simulink model "motor_1_2_3"  (R2023a)
settings: Solver=ode15s  StartTime=0.0  StopTime=sim_end_time  MaxStep=sim_max_step  RelTol=1e-3
values from neighbouring files (symbols this model uses):
  alpha_cu = 3.9 *10^-3    (= 0.0039)    [BLDC_Motor_params_03.m]    (also in DC_Motor_params_01.m; DC_Motor_params_02.m; DC_Motor_params_04.m; DC_Motor_params_05.m)
  b_m1 = .01    (= 0.01)    [DC_Motor_params_01.m]
  b_m2 = .01    (= 0.01)    [DC_Motor_params_02.m]
  b_m3 = .001    (= 0.001)    [BLDC_Motor_params_03.m]
  C_t1 = 19.57    [DC_Motor_params_01.m]
  C_t2 = 66.49    [DC_Motor_params_02.m]
  C_t3 = 50    [BLDC_Motor_params_03.m]
  ENABLE_SATURATIONS = 1    [run_flags.m]
  ENABLE_SENSORS = 1    [run_flags.m]
  enc_ppr_1 = 1024    [DC_Motor_params_01.m]
  enc_ppr_2 = 1024    [DC_Motor_params_02.m]
  filter_RC = 1/(max_freq*2*pi)    (= 0.00795774715459)    [filter_params.m]
  J_eq1 = J_1 + 1/8 * m_1 * d_1^2 / r_1^2    [DC_Motor_params_01.m]
  J_eq2 = J_2 + 1/8 * m_2 * d_2^2 / r_2^2    [DC_Motor_params_02.m]
  J_eq3 = J_3 + 1/8 * m_3 * d_3^2 / r_3^2    [BLDC_Motor_params_03.m]
  K_d1 = 0.022261    [PID_tuning.m]
  K_d2 = 0.07064    [PID_tuning.m]
  K_d3 = 0    [PID_tuning.m]
  k_e1 = 0.25    [DC_Motor_params_01.m]
  k_e2 = 0.56    [DC_Motor_params_02.m]
  k_e3 = 0.3    [BLDC_Motor_params_03.m]
  K_i1 = 0    [PID_tuning.m]
  K_i2 = 0    [PID_tuning.m]
  K_i3 = 0.4131    [PID_tuning.m]
  K_p1 = 6.6674    [PID_tuning.m]
  K_p2 = 15.5368    [PID_tuning.m]
  K_p3 = 0    [PID_tuning.m]
  k_t1 = 0.25    [DC_Motor_params_01.m]
  k_t2 = 0.56    [DC_Motor_params_02.m]
  k_t3 = 0.3    [BLDC_Motor_params_03.m]
  L_a1 = 7.5*10^-3    (= 0.0075)    [DC_Motor_params_01.m]
  L_a2 = 3*10^-3    (= 0.003)    [DC_Motor_params_02.m]
  L_a3 = 5*10^-3    (= 0.005)    [BLDC_Motor_params_03.m]
  r_1 = 25    [DC_Motor_params_01.m]
  r_2 = 5    [DC_Motor_params_02.m]
  r_3 = 2    [BLDC_Motor_params_03.m]
  r_a1_20 = 0.5    [DC_Motor_params_01.m]
  r_a2_20 = 0.25    [DC_Motor_params_02.m]
  r_a3_20 = 0.35    [BLDC_Motor_params_03.m]
  res_term_1 = 9.58    [DC_Motor_params_01.m]
  res_term_2 = 3.15    [DC_Motor_params_02.m]
  res_term_3 = 0.1    [BLDC_Motor_params_03.m]
  sampling_frequency = 40    [filter_params.m]
  T_s0_1 = 20    [use_machine_1.m]    (also in use_solo_motor_1.m)
  T_s0_2 = 20    [use_machine_1.m]    (also in use_solo_motor_2.m)
  T_s0_3 = 20    [use_machine_1.m]    (also in use_solo_motor_3.m)
  theta_m0_1 = 0    [use_machine_1.m]    (also in use_solo_motor_1.m)
  theta_m0_2 = 0    [use_machine_1.m]    (also in use_solo_motor_2.m = 3.14159265359)
  voltage_1 = 12    [DC_Motor_params_01.m]
  voltage_2 = 110    [DC_Motor_params_02.m]
  voltage_3 = 220    [BLDC_Motor_params_03.m]
libraries: slpidlib x1
settings Model: Creator=Usuario  LastModifiedBy=Usuario
settings DataIOCC: ExternalInput=[sim_t, sim_data_in]  LoadExternalInput=on

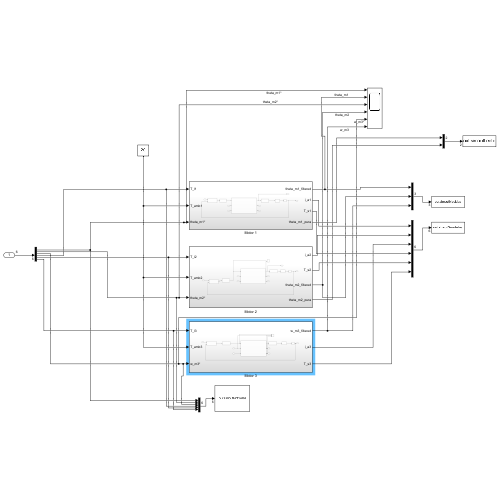
[thumbnail: Simulink's stored preview of the top-level diagram]
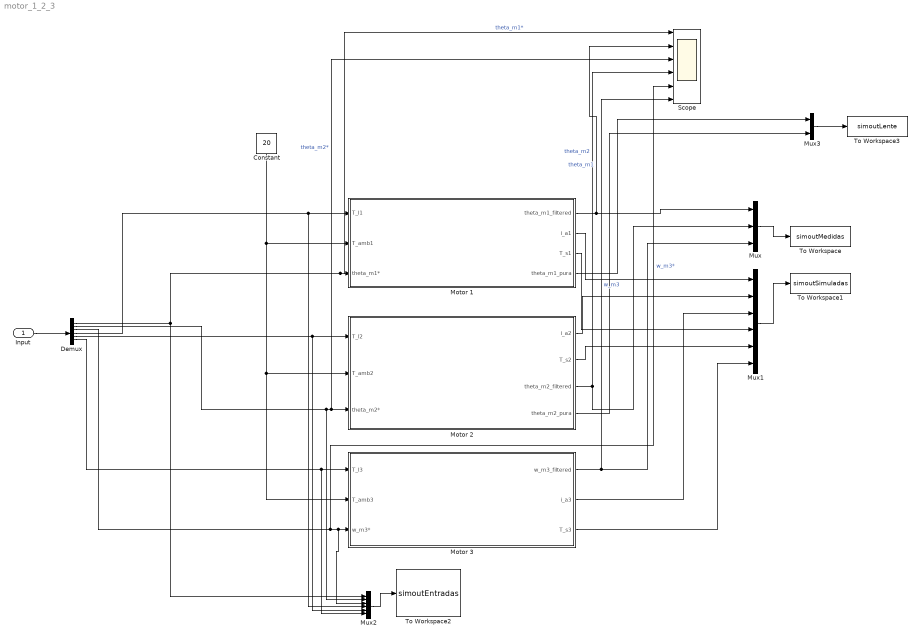
== system motor_1_2_3 ==
  Input : Inport
  Constant : Constant  Value=20
  Demux : Demux  Outputs=6
  Motor 1 : Subsystem
  Motor 2 : Subsystem
  Motor 3 : Subsystem
  Mux : Mux  Inputs=3
  Mux1 : Mux  Inputs=6
  Mux2 : Mux  Inputs=6
  Mux3 : Mux  Inputs=2
  Scope : Scope  NumInputPorts=6
  To Workspace : ToWorkspace  VariableName=simoutMedidas  SaveFormat=Timeseries  SampleTime=-1
  To Workspace1 : ToWorkspace  VariableName=simoutSimuladas  SaveFormat=Timeseries  SampleTime=-1
  To Workspace2 : ToWorkspace  VariableName=simoutEntradas  SaveFormat=Timeseries  SampleTime=-1
  To Workspace3 : ToWorkspace  VariableName=simoutLente  SaveFormat=Timeseries  SampleTime=-1
  wires:
  Constant/1 -> Motor 3/2(T_amb3), Motor 2/2(T_amb2), Motor 1/2(T_amb1)
  Input/1 -> Demux/1
  Demux/2 -> Mux2/2, Scope/3, Motor 2/3(theta_m2*)  "theta_m2*"
  Demux/3 -> Scope/5, Mux2/3, Motor 3/3(w_m3*)  "w_m3*"
  Demux/4 -> Mux2/4, Motor 1/1(T_l1)
  Demux/5 -> Mux2/5, Motor 2/1(T_l2)
  Demux/6 -> Mux2/6, Motor 3/1(T_l3)
  Demux/1 -> Scope/1, Motor 1/3(theta_m1*), Mux2/1  "theta_m1*"
  Motor 2/3(theta_m2_filtered) -> Mux/2, Scope/4  "theta_m2"
  Motor 3/1(w_m3_filtered) -> Scope/6, Mux/3  "w_m3"
  Motor 1/2(i_a1) -> Mux1/1
  Motor 2/1(i_a2) -> Mux1/2
  Motor 3/2(i_a3) -> Mux1/3
  Motor 1/3(T_s1) -> Mux1/4
  Motor 2/2(T_s2) -> Mux1/5
  Motor 3/3(T_s3) -> Mux1/6
  Mux/1 -> To Workspace/1
  Mux1/1 -> To Workspace1/1
  Motor 1/1(theta_m1_filtered) -> Scope/2, Mux/1  "theta_m1"
  Mux2/1 -> To Workspace2/1
  Mux3/1 -> To Workspace3/1
  Motor 1/4(theta_m1_pura) -> Mux3/1
  Motor 2/4(theta_m2_pura) -> Mux3/2

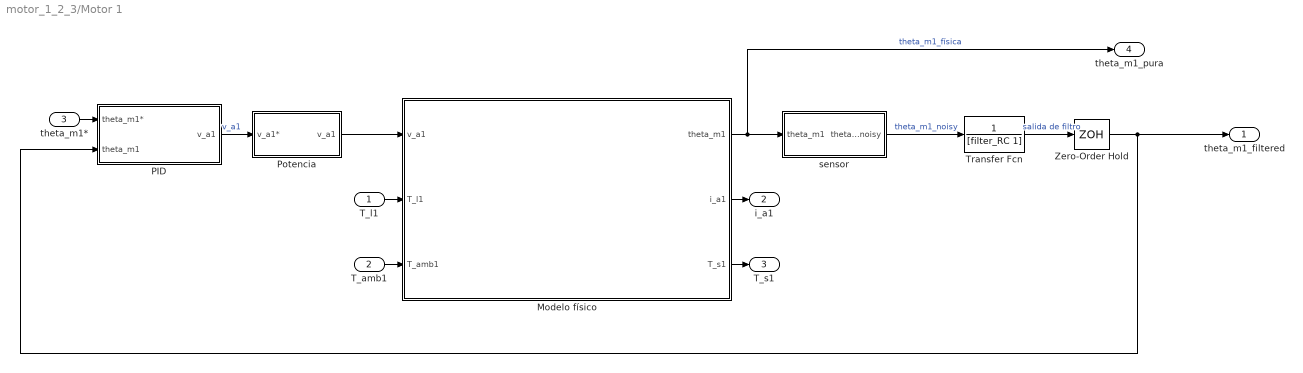
== system motor_1_2_3/Motor 1 ==
  T_l1 : Inport
  T_amb1 : Inport  Port=2
  theta_m1* : Inport  Port=3
  Modelo físico : Subsystem
  PID : Subsystem
  Potencia : Subsystem
  Transfer Fcn : TransferFcn  Denominator=[filter_RC 1]
  Zero-Order Hold : ZeroOrderHold  SampleTime=1/sampling_frequency
  sensor : Subsystem
  theta_m1_filtered : Outport  PortDimensions=1
  i_a1 : Outport  Port=2  PortDimensions=1
  T_s1 : Outport  Port=3  PortDimensions=1
  theta_m1_pura : Outport  Port=4
  wires:
  Modelo físico/1(theta_m1) -> theta_m1_pura/1, sensor/1(theta_m1)  "theta_m1_física"
  theta_m1*/1 -> PID/1(theta_m1*)
  Zero-Order Hold/1 -> PID/2(theta_m1), theta_m1_filtered/1
  sensor/1(theta_m1_noisy) -> Transfer Fcn/1  "theta_m1_noisy"
  Potencia/1(v_a1) -> Modelo físico/1(v_a1)
  Modelo físico/2(i_a1) -> i_a1/1
  Modelo físico/3(T_s1) -> T_s1/1
  T_amb1/1 -> Modelo físico/3(T_amb1)
  T_l1/1 -> Modelo físico/2(T_l1)
  PID/1(v_a1) -> Potencia/1(v_a1*)  "v_a1"
  Transfer Fcn/1 -> Zero-Order Hold/1  "salida de filtro"

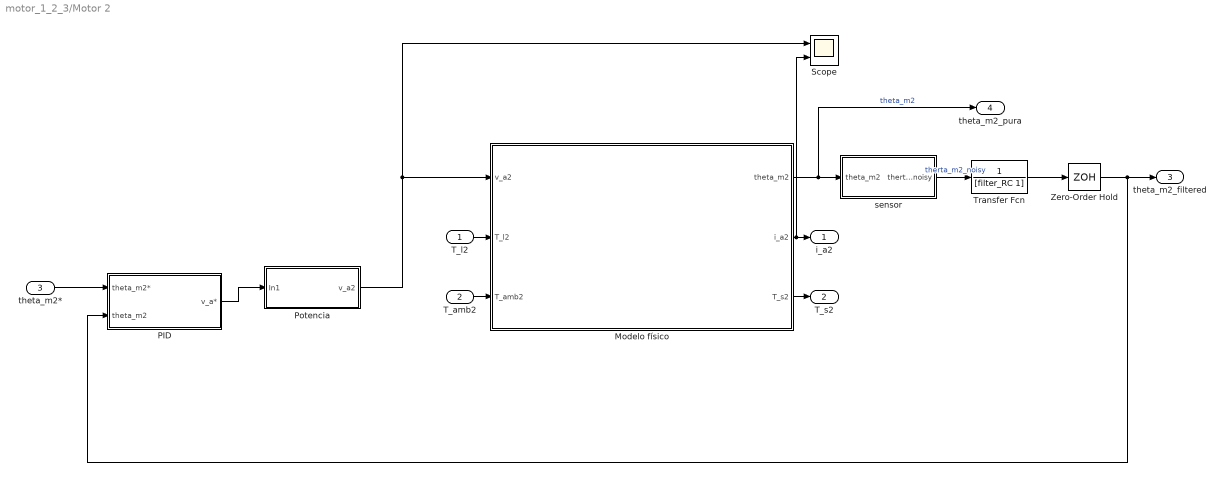
== system motor_1_2_3/Motor 2 ==
  T_l2 : Inport
  T_amb2 : Inport  Port=2
  theta_m2* : Inport  Port=3
  Modelo físico : Subsystem
  PID : Subsystem
  Potencia : Subsystem
  Scope : Scope  NumInputPorts=2
  Transfer Fcn : TransferFcn  Denominator=[filter_RC 1]
  Zero-Order Hold : ZeroOrderHold  SampleTime=1/sampling_frequency
  sensor : Subsystem
  i_a2 : Outport  PortDimensions=1
  T_s2 : Outport  Port=2  PortDimensions=1
  theta_m2_filtered : Outport  Port=3  PortDimensions=1
  theta_m2_pura : Outport  Port=4
  wires:
  sensor/1(therta_m2_noisy) -> Transfer Fcn/1  "therta_m2_noisy"
  Modelo físico/2(i_a2) -> Scope/2, i_a2/1
  Zero-Order Hold/1 -> theta_m2_filtered/1, PID/2(theta_m2)
  T_amb2/1 -> Modelo físico/3(T_amb2)
  T_l2/1 -> Modelo físico/2(T_l2)
  Potencia/1(v_a2) -> Scope/1, Modelo físico/1(v_a2)
  theta_m2*/1 -> PID/1(theta_m2*)
  Modelo físico/3(T_s2) -> T_s2/1
  PID/1(v_a*) -> Potencia/1(In1)
  Modelo físico/1(theta_m2) -> theta_m2_pura/1, sensor/1(theta_m2)  "theta_m2"
  Transfer Fcn/1 -> Zero-Order Hold/1

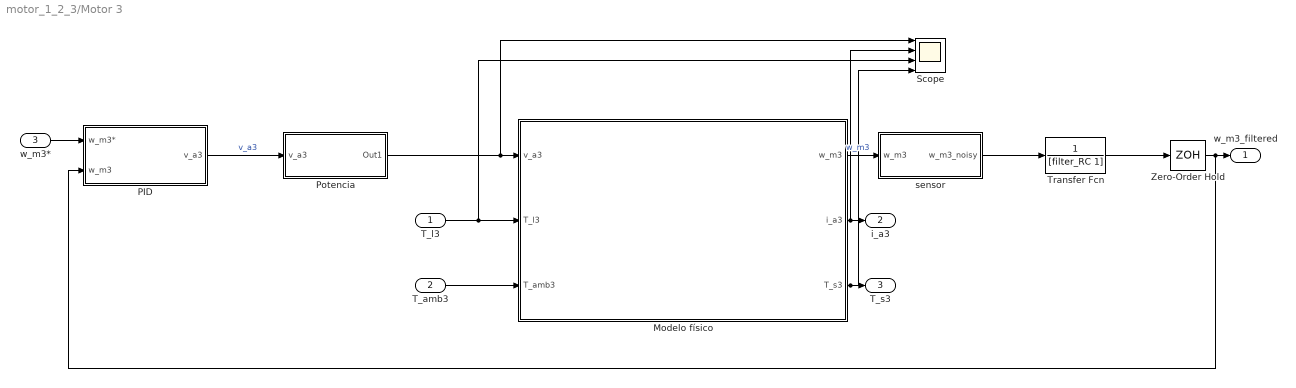
== system motor_1_2_3/Motor 3 ==
  T_l3 : Inport
  T_amb3 : Inport  Port=2
  w_m3* : Inport  Port=3
  Modelo físico : Subsystem
  PID : Subsystem
  Potencia : Subsystem
  Scope : Scope  NumInputPorts=4
  Transfer Fcn : TransferFcn  Denominator=[filter_RC 1]
  Zero-Order Hold : ZeroOrderHold  SampleTime=1/sampling_frequency
  sensor : Subsystem
  w_m3_filtered : Outport
  i_a3 : Outport  Port=2
  T_s3 : Outport  Port=3
  wires:
  PID/1(v_a3) -> Potencia/1(v_a3)  "v_a3"
  T_amb3/1 -> Modelo físico/3(T_amb3)
  sensor/1(w_m3_noisy) -> Transfer Fcn/1
  Potencia/1(Out1) -> Scope/1, Modelo físico/1(v_a3)
  T_l3/1 -> Scope/3, Modelo físico/2(T_l3)
  Modelo físico/1(w_m3) -> sensor/1(w_m3)  "w_m3"
  Modelo físico/3(T_s3) -> Scope/4, T_s3/1
  Zero-Order Hold/1 -> PID/2(w_m3), w_m3_filtered/1
  Modelo físico/2(i_a3) -> Scope/2, i_a3/1
  w_m3*/1 -> PID/1(w_m3*)
  Transfer Fcn/1 -> Zero-Order Hold/1

== system motor_1_2_3/Motor 1/Modelo físico ==
  v_a1 : Inport
  T_l1 : Inport  Port=2
  T_amb1 : Inport  Port=3
  Subsistema electromagnético : Subsystem
  Subsistema mecánico : Subsystem
  Subsistema térmico : Subsystem
  theta_m1 : Outport
  i_a1 : Outport  Port=2  PortDimensions=1
  T_s1 : Outport  Port=3  PortDimensions=1
  wires:
  Subsistema electromagnético/1(i_a1) -> Subsistema térmico/1(i_a1), Subsistema mecánico/1(i_a1), i_a1/1
  v_a1/1 -> Subsistema electromagnético/1(v_a1)
  T_l1/1 -> Subsistema mecánico/2(T_l1)
  T_amb1/1 -> Subsistema térmico/2(T_amb1)
  Subsistema térmico/1(T_s1) -> T_s1/1
  Subsistema térmico/2(r_a1) -> Subsistema electromagnético/2(r_a1)
  Subsistema mecánico/1(w_m1) -> Subsistema electromagnético/3(w_m1)
  Subsistema mecánico/2(theta_m1) -> theta_m1/1

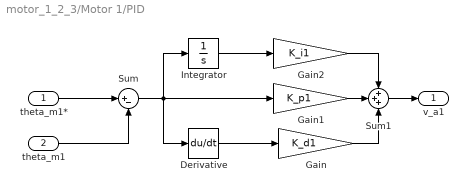
== system motor_1_2_3/Motor 1/PID ==
  theta_m1* : Inport
  theta_m1 : Inport  Port=2
  Derivative : Derivative
  Gain : Gain  Gain=K_d1
  Gain1 : Gain  Gain=K_p1
  Gain2 : Gain  Gain=K_i1
  Integrator : Integrator
  Sum : Sum  Inputs=|+-
  Sum1 : Sum  Inputs=+++
  v_a1 : Outport
  wires:
  theta_m1*/1 -> Sum/1
  theta_m1/1 -> Sum/2
  Sum/1 -> Integrator/1, Gain1/1, Derivative/1
  Integrator/1 -> Gain2/1
  Derivative/1 -> Gain/1
  Gain1/1 -> Sum1/2
  Gain2/1 -> Sum1/1
  Sum1/1 -> v_a1/1
  Gain/1 -> Sum1/3

== system motor_1_2_3/Motor 1/Potencia ==
  v_a1* : Inport
  Gain : Gain  Gain=ENABLE_SATURATIONS
  Gain1 : Gain  Gain=1-ENABLE_SATURATIONS
  Saturation : Saturate  UpperLimit=+voltage_1  LowerLimit=-voltage_1
  Sum : Sum  Inputs=|++
  v_a1 : Outport
  wires:
  v_a1*/1 -> Gain1/1, Saturation/1
  Saturation/1 -> Gain/1
  Gain/1 -> Sum/1
  Sum/1 -> v_a1/1
  Gain1/1 -> Sum/2

== system motor_1_2_3/Motor 1/sensor ==
  theta_m1 : Inport
  Gain : Gain  Gain=ENABLE_SENSORS
  Gain1 : Gain  Gain=1-ENABLE_SENSORS
  Scope : Scope  NumInputPorts=2
  Sum : Sum  Inputs=++|
  ruido de cuantización : Quantizer  QuantizationInterval=360/enc_ppr_1*(pi/180)
  theta_m1_noisy : Outport
  wires:
  Gain/1 -> Sum/2
  Gain1/1 -> Sum/1
  ruido de cuantización/1 -> Gain/1, Scope/1
  theta_m1/1 -> Gain1/1, ruido de cuantización/1, Scope/2
  Sum/1 -> theta_m1_noisy/1

== system motor_1_2_3/Motor 2/Modelo físico ==
  v_a2 : Inport
  T_l2 : Inport  Port=2
  T_amb2 : Inport  Port=3
  Subsistema electromagnético : Subsystem
  Subsistema mecánico : Subsystem
  Subsistema térmico : Subsystem
  theta_m2 : Outport
  i_a2 : Outport  Port=2  PortDimensions=1
  T_s2 : Outport  Port=3  PortDimensions=1
  wires:
  Subsistema electromagnético/1(i_a2) -> Subsistema térmico/1(i_a2), Subsistema mecánico/1(i_a2), i_a2/1
  v_a2/1 -> Subsistema electromagnético/1(v_a2)
  T_l2/1 -> Subsistema mecánico/2(T_l2)
  T_amb2/1 -> Subsistema térmico/2(T_amb2)
  Subsistema térmico/1(T_s2) -> T_s2/1
  Subsistema térmico/2(r_a2) -> Subsistema electromagnético/2(r_a2)
  Subsistema mecánico/1(w_m2) -> Subsistema electromagnético/3(w_m2)
  Subsistema mecánico/2(theta_m2) -> theta_m2/1

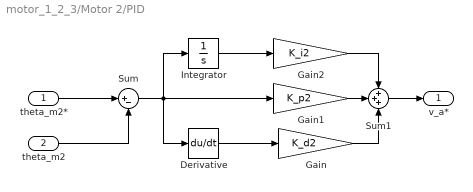
== system motor_1_2_3/Motor 2/PID ==
  theta_m2* : Inport
  theta_m2 : Inport  Port=2
  Derivative : Derivative
  Gain : Gain  Gain=K_d2
  Gain1 : Gain  Gain=K_p2
  Gain2 : Gain  Gain=K_i2
  Integrator : Integrator
  Sum : Sum  Inputs=|+-
  Sum1 : Sum  Inputs=+++
  v_a* : Outport
  wires:
  theta_m2*/1 -> Sum/1
  theta_m2/1 -> Sum/2
  Sum/1 -> Integrator/1, Gain1/1, Derivative/1
  Integrator/1 -> Gain2/1
  Derivative/1 -> Gain/1
  Gain1/1 -> Sum1/2
  Gain2/1 -> Sum1/1
  Sum1/1 -> v_a*/1
  Gain/1 -> Sum1/3

== system motor_1_2_3/Motor 2/Potencia ==
  In1 : Inport
  Gain : Gain  Gain=ENABLE_SATURATIONS
  Gain1 : Gain  Gain=1-ENABLE_SATURATIONS
  Saturation : Saturate  UpperLimit=+voltage_2  LowerLimit=-voltage_2
  Sum : Sum  Inputs=++|
  v_a2 : Outport
  wires:
  Saturation/1 -> Sum/2
  Gain/1 -> Saturation/1
  In1/1 -> Gain1/1, Gain/1
  Sum/1 -> v_a2/1
  Gain1/1 -> Sum/1

== system motor_1_2_3/Motor 2/sensor ==
  theta_m2 : Inport
  Gain : Gain  Gain=ENABLE_SENSORS
  Gain1 : Gain  Gain=1-ENABLE_SENSORS
  Scope : Scope  NumInputPorts=2
  Sum : Sum  Inputs=++|
  ruido de cuantización : Quantizer  QuantizationInterval=360/enc_ppr_2*(pi/180)
  therta_m2_noisy : Outport
  wires:
  Gain/1 -> Sum/2
  Gain1/1 -> Sum/1
  ruido de cuantización/1 -> Gain/1, Scope/1
  theta_m2/1 -> Gain1/1, ruido de cuantización/1, Scope/2
  Sum/1 -> therta_m2_noisy/1

== system motor_1_2_3/Motor 3/Modelo físico ==
  v_a3 : Inport
  T_l3 : Inport  Port=2
  T_amb3 : Inport  Port=3
  Subsistema electromagnético : Subsystem
  Subsistema mecánico : Subsystem
  Subsistema térmico : Subsystem
  w_m3 : Outport  PortDimensions=1
  i_a3 : Outport  Port=2  PortDimensions=1
  T_s3 : Outport  Port=3  PortDimensions=1
  wires:
  Subsistema electromagnético/1(i_a3) -> Subsistema térmico/1(i_a3), Subsistema mecánico/1(i_a3), i_a3/1
  v_a3/1 -> Subsistema electromagnético/1(v_a3)
  T_l3/1 -> Subsistema mecánico/2(T_l3)
  Subsistema mecánico/1(w_m3) -> w_m3/1, Subsistema electromagnético/3(w_m3)
  T_amb3/1 -> Subsistema térmico/2(T_amb3)
  Subsistema térmico/1(T_s3) -> T_s3/1
  Subsistema térmico/2(r_a3) -> Subsistema electromagnético/2(r_a3)

== system motor_1_2_3/Motor 3/PID ==
  w_m3* : Inport
  w_m3 : Inport  Port=2
  PID Controller : slpidlib/PID Controller  Controller=PID  Form=Parallel  TimeDomain=Continuous-time  UseExternalTs=off  SampleTime=-1  IntegratorMethod=Forward Euler  FilterMethod=Forward Euler  ControllerParametersSource=internal  P=K_p3  I=K_i3  UseKiTs=off  D=K_d3  N=100  UseFilter=on  TunerSelectOption=Transfer Function Based (PID Tuner App)  InitialConditionSource=internal  InitialConditionForIntegrator=0  InitialConditionForFilter=0  DifferentiatorICPrevScaledInput=0  ExternalReset=none  TrackingMode=off  Kt=1  LimitOutput=on  SatLimitsSource=internal  UpperSaturationLimit=voltage_3  LowerSaturationLimit=-voltage_3  LinearizeAsGain=on  AntiWindupMode=back-calculation  Kb=K_i3  LimitIntegrator=off  UpperIntegratorSaturationLimit=inf  LowerIntegratorSaturationLimit=-inf  POutMin=[]  POutMax=[]  IOutMin=[]  IOutMax=[]  DOutMin=[]  DOutMax=[]  NOutMin=[]  NOutMax=[]  SumOutMin=[]  SumOutMax=[]  SaturationOutMin=[]  SaturationOutMax=[]  PParamMin=[]  PParamMax=[]  IParamMin=[]  IParamMax=[]  DParamMin=[]  DParamMax=[]  NParamMin=[]  NParamMax=[]  KbParamMin=[]  KbParamMax=[]  KtParamMin=[]  KtParamMax=[]  KbOutMin=[]  KbOutMax=[]  KtOutMin=[]  KtOutMax=[]  IntegratorOutMin=[]  IntegratorOutMax=[]  FilterOutMin=[]  FilterOutMax=[]  SumI1OutMin=[]  SumI1OutMax=[]  SumI2OutMin=[]  SumI2OutMax=[]  SumI3OutMin=[]  SumI3OutMax=[]  SumI4OutMin=[]  SumI4OutMax=[]  SumDOutMin=[]  SumDOutMax=[]  DifferentiatorOutMin=[]  DifferentiatorOutMax=[]  FilterDiffOutCoefMin=[]  FilterDiffOutCoefMax=[]  ReciprocalOutMin=[]  ReciprocalOutMax=[]  SumDenOutMin=[]  SumDenOutMax=[]  SumNumOutMin=[]  SumNumOutMax=[]  DivideOutMin=[]  DivideOutMax=[]  UdiffTsProdOutMin=[]  UdiffTsProdOutMax=[]  NTsProdOutMin=[]  NTsProdOutMax=[]  UintegralTsProdOutMin=[]  UintegralTsProdOutMax=[]  UngainTsProdOutMin=[]  UngainTsProdOutMax=[]  ClampingZeroOutDataTypeStr=Inherit: Inherit via back propagation  ClampingZeroOutMin=[]  ClampingZeroOutMax=[]  FilterDenConstantOutDataTypeStr=Inherit: Inherit via back propagation  FilterDenConstantOutMin=[]  FilterDenConstantOutMax=[]  PCopyOutDataTypeStr=Inherit: Inherit via back propagation  PCopyOutMin=[]  PCopyOutMax=[]  NCopyOutDataTypeStr=Inherit: Inherit via back propagation  NCopyOutMin=[]  NCopyOutMax=[]  IntegratorContinuousStateAttributes=''  IntegratorStateMustResolveToSignalObject=off  IntegratorRTWStateStorageClass=Auto  FilterContinuousStateAttributes=''  FilterStateMustResolveToSignalObject=off  FilterRTWStateStorageClass=Auto  ParallelPVariant=InternalParameters  IdealPVariant=Disabled  IVariant=InternalParameters  DVariant=InternalParameters  IntegratorVariant=Continuous  SatVariant=Enabled  AWVariant=BackCalculation  PCopyVariant=Disabled  TRVariant=Disabled  FdbkBlocksVariant=Forward  IdealPFdbkVariant=Disabled  SatFdbkVariant=Disabled  DerivativeFilterVariant=ContFilter  NVariant=InternalParameters  NCopyVariant=Disabled  FilterICVariant=InternalICsFilter  IntegratorICVariant=InternalICs  ExternalResetVariant=Disabled  TRSumVariant=Passthrough  SumFdbkVariant=Disabled  SumVariant=Sum_PID  TsampFilterVariant=InternalTs  TsampNgainVariant=Passthrough  TsampIntegralVariant=Disabled_SignalSpec  ExternalSaturationOutDataTypeStr=Inherit: Same as second input
  Sum : Sum  Inputs=|+-
  v_a3 : Outport
  wires:
  w_m3*/1 -> Sum/1
  w_m3/1 -> Sum/2
  Sum/1 -> PID Controller/1
  PID Controller/1 -> v_a3/1

== system motor_1_2_3/Motor 3/Potencia ==
  v_a3 : Inport
  Gain : Gain  Gain=ENABLE_SATURATIONS
  Gain1 : Gain  Gain=1-ENABLE_SATURATIONS
  Saturation : Saturate  UpperLimit=+voltage_3  LowerLimit=-voltage_3
  Sum : Sum  Inputs=++|
  Out1 : Outport
  wires:
  v_a3/1 -> Gain1/1, Gain/1
  Saturation/1 -> Sum/2
  Gain/1 -> Saturation/1
  Sum/1 -> Out1/1
  Gain1/1 -> Sum/1

== system motor_1_2_3/Motor 3/sensor ==
  w_m3 : Inport
  Gain : Gain  Gain=1/(2*pi)
  Gain1 : Gain  Gain=(2*pi)
  Gain2 : Gain  Gain=ENABLE_SENSORS
  Gain3 : Gain  Gain=1-ENABLE_SENSORS
  Quantizer : Quantizer  QuantizationInterval=sensibilidad_sensor_3
  Scope : Scope  NumInputPorts=2
  Sum : Sum  Inputs=++|
  w_m3_noisy : Outport
  wires:
  w_m3/1 -> Gain3/1, Gain2/1
  Quantizer/1 -> Gain1/1, Scope/1
  Gain/1 -> Quantizer/1
  Gain1/1 -> Sum/2
  Gain2/1 -> Scope/2, Gain/1
  Gain3/1 -> Sum/1
  Sum/1 -> w_m3_noisy/1

== system motor_1_2_3/Motor 1/Modelo físico/Subsistema electromagnético ==
  v_a1 : Inport
  r_a1 : Inport  Port=2
  w_m1 : Inport  Port=3
  Gain1 : Gain  Gain=k_e1
  Gain2 : Gain  Gain=1/L_a1
  Integrator : Integrator
  Product : Product
  Sum : Sum  Inputs=-+-  OutMin=[1]  OutMax=[1]
  i_a1 : Outport
  wires:
  v_a1/1 -> Sum/2
  Integrator/1 -> Product/2, i_a1/1
  Product/1 -> Sum/1
  w_m1/1 -> Gain1/1
  Gain1/1 -> Sum/3
  Sum/1 -> Gain2/1
  Gain2/1 -> Integrator/1
  r_a1/1 -> Product/1

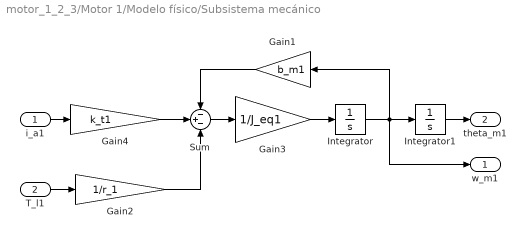
== system motor_1_2_3/Motor 1/Modelo físico/Subsistema mecánico ==
  i_a1 : Inport
  T_l1 : Inport  Port=2
  Gain1 : Gain  Gain=b_m1
  Gain2 : Gain  Gain=1/r_1
  Gain3 : Gain  Gain=1/J_eq1
  Gain4 : Gain  Gain=k_t1
  Integrator : Integrator
  Integrator1 : Integrator  InitialCondition=theta_m0_1
  Sum : Sum  Inputs=-+-
  w_m1 : Outport
  theta_m1 : Outport  Port=2
  wires:
  i_a1/1 -> Gain4/1
  Integrator/1 -> w_m1/1, Gain1/1, Integrator1/1
  Gain1/1 -> Sum/1
  T_l1/1 -> Gain2/1
  Gain3/1 -> Integrator/1
  Sum/1 -> Gain3/1
  Integrator1/1 -> theta_m1/1
  Gain2/1 -> Sum/3
  Gain4/1 -> Sum/2

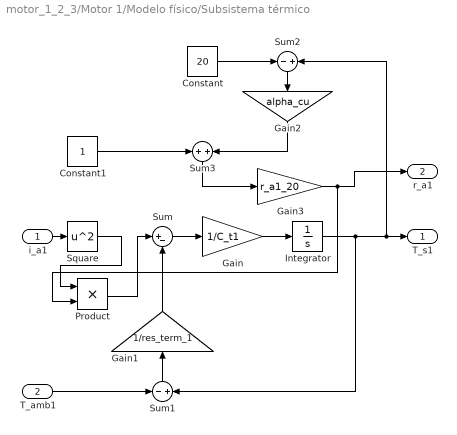
== system motor_1_2_3/Motor 1/Modelo físico/Subsistema térmico ==
  i_a1 : Inport
  T_amb1 : Inport  Port=2
  Constant : Constant  Value=20
  Constant1 : Constant
  Gain : Gain  Gain=1/C_t1
  Gain1 : Gain  Gain=1/res_term_1
  Gain2 : Gain  Gain=alpha_cu
  Gain3 : Gain  Gain=r_a1_20
  Integrator : Integrator  InitialCondition=T_s0_1
  Product : Product
  Square : Math  Operator=square
  Sum : Sum  Inputs=|+-
  Sum1 : Sum  Inputs=-|+
  Sum2 : Sum  Inputs=-|+
  Sum3 : Sum  Inputs=+|+
  T_s1 : Outport
  r_a1 : Outport  Port=2
  wires:
  i_a1/1 -> Square/1
  Sum3/1 -> Gain3/1
  Gain2/1 -> Sum3/2
  Square/1 -> Product/1
  Gain3/1 -> Product/2, r_a1/1
  Sum2/1 -> Gain2/1
  T_amb1/1 -> Sum1/1
  Constant1/1 -> Sum3/1
  Gain/1 -> Integrator/1
  Sum/1 -> Gain/1
  Integrator/1 -> Sum1/2, Sum2/2, T_s1/1
  Constant/1 -> Sum2/1
  Sum1/1 -> Gain1/1
  Gain1/1 -> Sum/2
  Product/1 -> Sum/1

== system motor_1_2_3/Motor 2/Modelo físico/Subsistema electromagnético ==
  v_a2 : Inport
  r_a2 : Inport  Port=2
  w_m2 : Inport  Port=3
  Gain1 : Gain  Gain=k_e2
  Gain2 : Gain  Gain=1/L_a2
  Integrator : Integrator
  Product : Product
  Sum : Sum  Inputs=-+-
  i_a2 : Outport
  wires:
  v_a2/1 -> Sum/2
  Integrator/1 -> Product/2, i_a2/1
  Product/1 -> Sum/1
  w_m2/1 -> Gain1/1
  Gain1/1 -> Sum/3
  Sum/1 -> Gain2/1
  Gain2/1 -> Integrator/1
  r_a2/1 -> Product/1

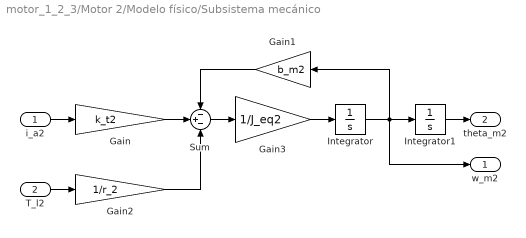
== system motor_1_2_3/Motor 2/Modelo físico/Subsistema mecánico ==
  i_a2 : Inport
  T_l2 : Inport  Port=2
  Gain : Gain  Gain=k_t2
  Gain1 : Gain  Gain=b_m2
  Gain2 : Gain  Gain=1/r_2
  Gain3 : Gain  Gain=1/J_eq2
  Integrator : Integrator
  Integrator1 : Integrator  InitialCondition=theta_m0_2
  Sum : Sum  Inputs=-+-
  w_m2 : Outport
  theta_m2 : Outport  Port=2
  wires:
  i_a2/1 -> Gain/1
  Gain/1 -> Sum/2
  Integrator/1 -> w_m2/1, Gain1/1, Integrator1/1
  Gain1/1 -> Sum/1
  T_l2/1 -> Gain2/1
  Gain3/1 -> Integrator/1
  Sum/1 -> Gain3/1
  Integrator1/1 -> theta_m2/1
  Gain2/1 -> Sum/3

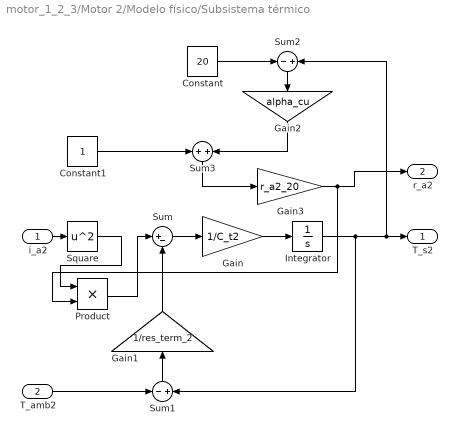
== system motor_1_2_3/Motor 2/Modelo físico/Subsistema térmico ==
  i_a2 : Inport
  T_amb2 : Inport  Port=2
  Constant : Constant  Value=20
  Constant1 : Constant
  Gain : Gain  Gain=1/C_t2
  Gain1 : Gain  Gain=1/res_term_2
  Gain2 : Gain  Gain=alpha_cu
  Gain3 : Gain  Gain=r_a2_20
  Integrator : Integrator  InitialCondition=T_s0_2
  Product : Product
  Square : Math  Operator=square
  Sum : Sum  Inputs=|+-
  Sum1 : Sum  Inputs=-|+
  Sum2 : Sum  Inputs=-|+
  Sum3 : Sum  Inputs=+|+
  T_s2 : Outport  PortDimensions=1
  r_a2 : Outport  Port=2
  wires:
  i_a2/1 -> Square/1
  Sum3/1 -> Gain3/1
  Gain2/1 -> Sum3/2
  Square/1 -> Product/1
  Gain3/1 -> Product/2, r_a2/1
  Sum2/1 -> Gain2/1
  T_amb2/1 -> Sum1/1
  Constant1/1 -> Sum3/1
  Gain/1 -> Integrator/1
  Sum/1 -> Gain/1
  Integrator/1 -> Sum1/2, Sum2/2, T_s2/1
  Constant/1 -> Sum2/1
  Sum1/1 -> Gain1/1
  Gain1/1 -> Sum/2
  Product/1 -> Sum/1

== system motor_1_2_3/Motor 3/Modelo físico/Subsistema electromagnético ==
  v_a3 : Inport
  r_a3 : Inport  Port=2
  w_m3 : Inport  Port=3
  Gain1 : Gain  Gain=k_e3
  Gain2 : Gain  Gain=1/L_a3
  Integrator : Integrator
  Product : Product
  Scope : Scope  NumInputPorts=3
  Sum : Sum  Inputs=-+-
  i_a3 : Outport  PortDimensions=1
  wires:
  v_a3/1 -> Scope/1, Sum/2  "v_a"
  Integrator/1 -> Product/2, i_a3/1
  Product/1 -> Scope/3, Sum/1  "caida de V por resistencia"
  w_m3/1 -> Gain1/1
  Gain1/1 -> Scope/2, Sum/3  "backfem"
  Sum/1 -> Gain2/1
  Gain2/1 -> Integrator/1
  r_a3/1 -> Product/1

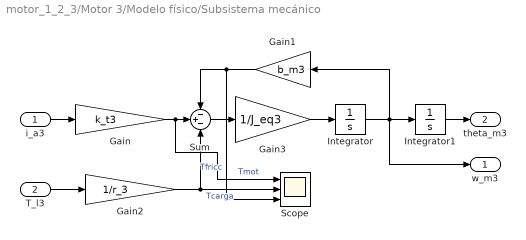
== system motor_1_2_3/Motor 3/Modelo físico/Subsistema mecánico ==
  i_a3 : Inport
  T_l3 : Inport  Port=2
  Gain : Gain  Gain=k_t3
  Gain1 : Gain  Gain=b_m3
  Gain2 : Gain  Gain=1/r_3
  Gain3 : Gain  Gain=1/J_eq3
  Integrator : Integrator
  Integrator1 : Integrator
  Scope : Scope  NumInputPorts=3
  Sum : Sum  Inputs=-+-
  w_m3 : Outport  PortDimensions=1
  theta_m3 : Outport  Port=2  PortDimensions=1
  wires:
  i_a3/1 -> Gain/1
  Gain/1 -> Scope/1, Sum/2  "Tmot"
  Integrator/1 -> w_m3/1, Gain1/1, Integrator1/1
  Gain1/1 -> Sum/1, Scope/3  "Tfricc"
  T_l3/1 -> Gain2/1
  Gain3/1 -> Integrator/1
  Sum/1 -> Gain3/1
  Integrator1/1 -> theta_m3/1
  Gain2/1 -> Scope/2, Sum/3  "Tcarga"

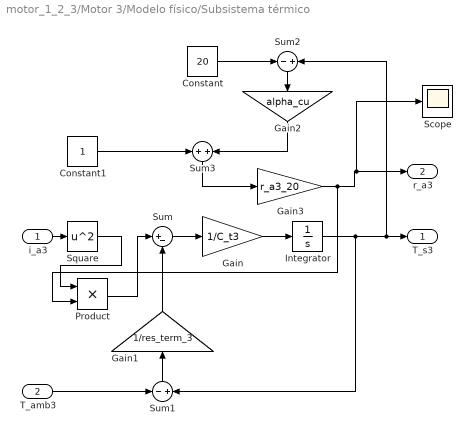
== system motor_1_2_3/Motor 3/Modelo físico/Subsistema térmico ==
  i_a3 : Inport
  T_amb3 : Inport  Port=2
  Constant : Constant  Value=20
  Constant1 : Constant
  Gain : Gain  Gain=1/C_t3
  Gain1 : Gain  Gain=1/res_term_3
  Gain2 : Gain  Gain=alpha_cu
  Gain3 : Gain  Gain=r_a3_20
  Integrator : Integrator  InitialCondition=T_s0_3
  Product : Product
  Scope : Scope
  Square : Math  Operator=square
  Sum : Sum  Inputs=|+-
  Sum1 : Sum  Inputs=-|+
  Sum2 : Sum  Inputs=-|+
  Sum3 : Sum  Inputs=+|+
  T_s3 : Outport  PortDimensions=1
  r_a3 : Outport  Port=2  PortDimensions=1
  wires:
  i_a3/1 -> Square/1
  Sum3/1 -> Gain3/1
  Gain2/1 -> Sum3/2
  Square/1 -> Product/1
  Gain3/1 -> Product/2, Scope/1, r_a3/1
  Sum2/1 -> Gain2/1
  T_amb3/1 -> Sum1/1
  Constant1/1 -> Sum3/1
  Gain/1 -> Integrator/1
  Sum/1 -> Gain/1
  Integrator/1 -> Sum1/2, Sum2/2, T_s3/1
  Constant/1 -> Sum2/1
  Sum1/1 -> Gain1/1
  Gain1/1 -> Sum/2
  Product/1 -> Sum/1
